simulink model "APP_MyApplication"  (R2018b)
settings: Solver=VariableStepDiscrete  StartTime=0.0  StopTime=10  RelTol=1e-3
PreLoadFcn:
  | if(exist('MBDS_ModelCallback', 'file')), MBDS_ModelCallback('PreLoad'); end;
PostLoadFcn:
  | if(exist('MBDS_ModelCallback', 'file')), MBDS_ModelCallback('PostLoad'); end;
InitFcn:
  | if(exist('MBDS_ModelCallback', 'file')), MBDS_ModelCallback('Init'); end;
StartFcn:
  | if(exist('MBDS_ModelCallback', 'file')), MBDS_ModelCallback('Start'); end;
StopFcn:
  | if(exist('MBDS_ModelCallback', 'file')), MBDS_ModelCallback('Stop'); end;
undefined symbols (not defined in the file): sigbuilder_block, Ts
libraries: KIBES_Signal x499, simulink x8
(part 1 of 10)
PreSaveFcn:
  | if(exist('MBDS_ModelCallback', 'file')), MBDS_ModelCallback('PreSave'); end;
CloseFcn:
  | if(exist('MBDS_ModelCallback', 'file')), MBDS_ModelCallback('Close'); end;
Description:
  | Design model of an MBDS Application
settings Model: IsTargetCode=true  MBDS_Version=08.20  Creator=Udo Kaiser (uidf0608)  LastModifiedBy=uidj2473
settings ConfigSet: Description=MBDS configuration set optimized for simulation of model designs for automotive embedded systems.
settings SolverCC: MinimalZcImpactIntegration=on
settings DataIOCC: MaxDataPoints=100  SaveFormat=StructureWithTime  SaveOutput=off  DSMLogging=off  VisualizeSimOutput=off  SaveTime=off  SignalLoggingName=LogSignals
settings OptimizationCC: UseDivisionForNetSlopeComputation=UseDivisionForReciprocalsOfIntegersOnly  UseFloatMulNetSlope=on  DefaultUnderspecifiedDataType=single  OptimizeBlockIOStorage=off  BufferReuse=off  GlobalBufferReuse=off  StrengthReduction=on  ExpressionFolding=off  ExpressionDepthLimit=2147483647  LocalBlockOutputs=off  EfficientFloat2IntCast=on  LifeSpan=inf  BufferReusableBoundary=off  OptimizeBlockOrder=speed  OptimizeDataStoreBuffers=off  BusAssignmentInplaceUpdate=off  LabelGuidedReuse=on
settings DebuggingCC: SignalInfNanChecking=error  AlgebraicLoopMsg=error  ArtificialAlgebraicLoopMsg=error  UnderspecifiedInitializationDetection=Classic  CheckExecutionContextPreStartOutputMsg=on  CheckExecutionContextRuntimeOutputMsg=on  BlockPriorityViolationMsg=error  MinStepSizeMsg=error  TimeAdjustmentMsg=warning  SolverPrmCheckMsg=error  InheritedTsInSrcMsg=none  SingleTaskRateTransMsg=error  TasksWithSamePriorityMsg=error  SigSpecEnsureSampleTimeMsg=error  CheckMatrixSingularityMsg=error  ParameterUnderflowMsg=error  ParameterTunabilityLossMsg=error  FixptConstUnderflowMsg=warning  FixptConstOverflowMsg=warning  FixptConstPrecisionLossMsg=warning  VectorMatrixConversionMsg=error  SignalLabelMismatchMsg=warning  SFcnCompatibilityMsg=error  FrameProcessingCompatibilityMsg=warning  UniqueDataStoreMsg=error  BusObjectLabelMismatch=error  RootOutportRequireBusObject=error  AllowSymbolicDim=off  ModelReferenceIOMsg=error  ModelReferenceIOMismatchMessage=error  UnknownTsInhSupMsg=error  ModelReferenceDataLoggingMessage=error  StateNameClashWarn=warning  SimStateOlderReleaseMsg=warning  StrictBusMsg=ErrorOnBusTreatedAsVector  NonBusSignalsTreatedAsBus=error  SFInvalidInputDataAccessInChartInitDiag=error  SFTransitionOutsideNaturalParentDiag=error  SFUnreachableExecutionPathDiag=error  SFUndirectedBroadcastEventsDiag=error  SFTransitionActionBeforeConditionDiag=error  SFTemporalDelaySmallerThanSampleTimeDiag=error  SFExecutionAtInitializationDiag=none
settings HardwareCC: ProdBitPerPointer=32  ProdBitPerSizeT=32  ProdBitPerPtrDiffT=32  ProdLargestAtomicInteger=Long  ProdEndianess=BigEndian  ProdWordSize=32  ProdLongLongMode=on  ProdHWDeviceType=Custom Processor  TargetHWDeviceType=32-bit Generic
settings ModelReferenceCC: PropagateSignalLabelsOutOfModel=off
settings SFSimCC: SimUseLocalCustomCode=off  SimGenImportedTypeDefs=on  CompileTimeRecursionLimit=0  EnableRuntimeRecursion=off  MATLABDynamicMemAlloc=off  DefaultCustomCodeFunctionArrayLayout=Column-major
settings RTWCC: SystemTargetFile=MBDS.tlc  GenCodeOnly=on  TemplateMakefile=MBDS.tmf  Description=MBDS Target  GenerateReport=on  RTWUseLocalCustomCode=off  IncludeHyperlinkInReport=on  LaunchReport=on  GenerateTraceReport=on  GenerateTraceReportSl=on  GenerateTraceReportSf=on  GenerateTraceReportEml=on  GenerateCodeMetricsReport=on  RTWCompilerOptimization=on
settings CodeAppCC: ForceParamTrailComments=on  IgnoreCustomStorageClasses=off  OperatorAnnotations=on  SimulinkDataObjDesc=on  SFDataObjDesc=on  MangleLength=2  CustomSymbolStrType=$N$R$M  CustomSymbolStrFcn=$R$M  CustomSymbolStrUtil=$n$C  InsertBlockDesc=on  StateflowObjectComments=on  MATLABSourceComments=on  ReqsInCode=on  UseSimReservedNames=on
settings STFCustomTargetCC: UtilityFuncGeneration=Shared location  MultiwordLength=256  DynamicStringBufferSize=2  InferredTypesCompatibility=on  ModelReferenceCompliant=off  IncludeMdlTerminateFcn=off  CombineOutputUpdateFcns=on  CombineSignalStateStructs=on  SuppressErrorStatus=on  ERTCustomFileBanners=on  SupportComplex=off  SupportContinuousTime=off  SupportNonInlinedSFcns=off  RemoveDisableFunc=on  RemoveResetFunc=on  ParenthesesLevel=Maximum  CastingMode=Standards  MATLABClassNameForMDSCustomization=Simulink.SoftwareTarget.ERTCustomization  GenerateSharedConstants=off  SystemTargetFile=MBDS.tlc
settings ERTTargetCC: UtilityFuncGeneration=Shared location  DynamicStringBufferSize=2  InferredTypesCompatibility=on  ModelReferenceCompliant=off  ParMdlRefBuildCompliant=off  CompOptLevelCompliant=off  ConcurrentExecutionCompliant=off  IncludeMdlTerminateFcn=off  CombineSignalStateStructs=on  SuppressErrorStatus=on  SupportComplex=off  RemoveDisableFunc=on  ParenthesesLevel=Maximum  CastingMode=Standards  ModelStepFunctionPrototypeControlCompliant=off  CPPClassGenCompliant=off  UseToolchainInfoCompliant=off  GenerateSharedConstants=off  ERTCustomFileTemplate=example_file_process.tlc  EnableDataOwnership=on  PreserveExpressionOrder=on  PreserveIfCondition=on  SuppressUnreachableDefaultCases=off  EnableSignedLeftShifts=off  EnableSignedRightShifts=off  IndentStyle=Allman  NewlineStyle=CR+LF
settings ConfigComp: CovScope=ReferencedModels  CovIncludeTopModel=off  CovPath=APP_MyApplication/Model/APP_MyApplication_  CovSaveName=covData  CovMetricSettings=dsw  CovFilter=MBDS_CoverageFilter  CovHTMLOptions=-sRT=1 -sVT=0 -aTS=1 -bRG=1 -bTC=1 -hTR=1 -nFC=0 -nFD=0 -scm=1 -bcm=1 -xEv=0 -xEM=1  CovHtmlReporting=on  CovSaveOutputData=off  CovDataFileName=covData  CovShowResultsExplorer=off  CovExternalEMLEnable=off  CovSFcnEnable=off

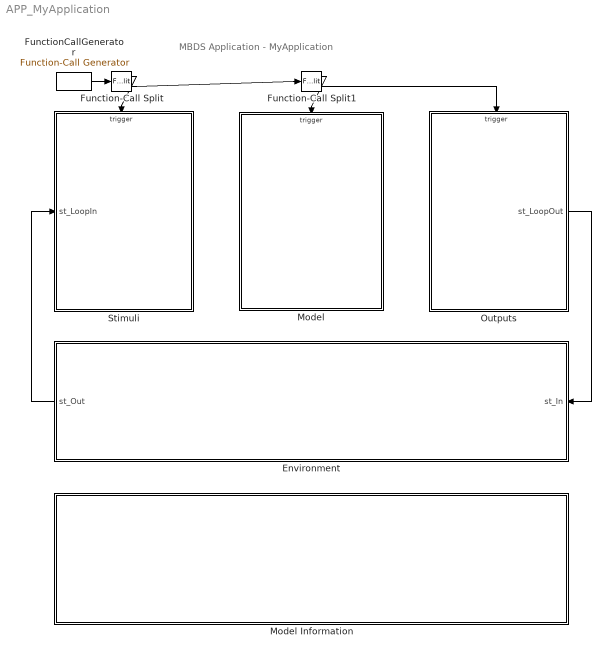
== system APP_MyApplication ==
  note: MBDS Application - MyApplication
  Environment : Subsystem  Description=Environment subsystem for a MBDS model.
  Function-Call Split : FunctionCallSplit  InitFcn=|  NumOutputPorts=2
      | try
      |    MBDS_BlockCallback('Update', gcb);
      | end
      | try
      |    MBDS_BlockCallback('Update', gcb);
      | end
  Function-Call Split1 : FunctionCallSplit  InitFcn=|  NumOutputPorts=2
      | try
      |    MBDS_BlockCallback('Update', gcb);
      | end
      | try
      |    MBDS_BlockCallback('Update', gcb);
      | end
  FunctionCallGenerator : simulink/Ports & Subsystems/Function-Call Generator  sample_time=0.05  numberOfIterations=1
      settings: AttributesFormatString=Ts = %<sample_time>
  Model : Subsystem  Description=Model subsystem for a MBDS model. Here, the input signals to the model functionality are resolved from the Stimuli bus and the output signals of the model functionality are summarized into the Results bus.
  Model Information : Subsystem  InitFcn=|  mask(ModelInformation){MBDS_LibraryBlock=on, Company=-, Department=-, Responsible=-, Status=In Work, Complete=on, Check=on, Test=on, Optimize=on, Documentation=on, FcnErrors=off, GenericToDo=off, DocumentState=Draft, GenericToDoName=Enter a user specific ToDo text, MBDS_BlockVersion=07.00}
      | if(exist('MBDS_BlockCallback', 'file'))
      |    MBDS_BlockCallback('Update', gcb);
      | end
      mask prompts: MBDS_LibraryBlock "MBDS Library Block"; Complete "Complete Implementation"; Check "Check Modelling Guidelines"; Test "Test Functionality"; Optimize "Optimize Implementation"; Documentation "Create Documentation"; FcnErrors "Remove Functional Errors"; GenericToDo "Enter a user specific ToDo text"; DocumentState "Document State:"; GenericToDoName "Generic ToDo Name:"; MBDS_BlockVersion "Block version:"
      mask help: This block displays model information and ToDo's on it's block mask. Via the block parameter mask further model information and configuration options can be accessed.
      mask init:
      | if(exist('MBDS_BlockCallback', 'file'))
      |    MBDS_BlockCallback('Copy', gcb);    
      | end
      mask Help: eval(['open([workdir(''library_dir:''),''\Blockset\help\'',get_param(gcb,''MaskType''),''.html''])'])
      mask TypeOptions Status: In Work | Done
      mask TypeOptions DocumentState: Draft | Final | Released
      mask Callback GenericToDoName:
      | MaskPrompts = get_param(gcb, 'MaskPrompts');
      | MaskPrompts{12} = get_param(gcb, 'GenericToDoName');
      | if(length(MaskPrompts{12}) > 75)
      |    MaskPrompts{12} = MaskPrompts{12}(1:75);
      |    set_param(gcb, 'GenericToDoName', MaskPrompts{12});
      | end
      | set_param(gcb, 'MaskPrompts', MaskPrompts);
      | clear MaskPrompts;
      mask DialogControl ParameterTabVar0 Prompt: Info
      mask DialogControl ParameterTabVar01 Prompt: ToDo's
      mask DialogControl ParameterTabVar012 Prompt: Options
      mask DialogControl ParameterTabVar0123 Prompt: Version
      mask Display:
      | % Get ToDo's
      | IsComplete       = strcmpi(Complete, 'on');
      | IsOptimize       = strcmpi(Optimize, 'on');
      | IsCheck          = strcmpi(Check, 'on');
      | IsDocumentation  = strcmpi(Documentation, 'on');
      | IsTest           = strcmpi(Test, 'on');
      | IsFcnErrors      = strcmpi(FcnErrors, 'on');
      | IsGenericToDo    = strcmpi(GenericToDo, 'on');
      | 
      | % Determine status
      | if(IsFcnErrors || IsTest || IsComplete || IsDocumentation || IsCheck || IsOptimize || IsGenericToDo)
      |    Status = 'In Work';
      | else
      |    Status = 'Done';
      | end
      | 
      | % Update status parameter
      | if(~strcmpi(get_param(gcb, 'Status'), Status))
      |    set_param(gcb, 'Status', Status);
      | end
      | 
      | % Determine severity
      | if(IsFcnErrors)
      |    % Severity: Critical
      |    BoxColorFile = 'Box_Red.tif';
      |    IconFile     = 'State_Red.jpg';
      | elseif (IsTest || IsComplete || IsGenericToDo)
      |    % Severity: Major
      |    BoxColorFile = 'Box_Orange.tif';
      |    IconFile     = 'State_Orange.jpg';
      | elseif (IsDocumentation || IsCheck || IsOptimize)
      |    % Severity: Minor
      |    BoxColorFile = 'Box_Grey.tif';
      |    IconFile     = 'State_Grey.jpg';
      | else
      |    % Severity: None
      |    BoxColorFile = 'Box_Green.tif';
      |    IconFile     = 'State_Green.jpg';
      | end
      | 
      | % Display Model Information
      | InfoStr1 = sprintf('%s', get_param(bdroot, 'Name'));
      | InfoStr2 = sprintf('Model Version:  %s', get_param(bdroot, 'ModelVersion'));
      | InfoStr3 = sprintf('Company:  %s', Company);
      | InfoStr4 = sprintf('Department:  %s', Department);
      | InfoStr5 = sprintf('Responsible:  %s', Responsible);
      | InfoStr6 = sprintf('Last Modified by:  %s at %s', get_param(bdroot, 'LastModifiedBy'), get_param(bdroot, 'LastModifiedDate'));
      | %Y is to do!!!!
      | text(0.5, 0.69, sprintf('%s\n%s\n%s\n%s\n%s\n%s\n%s', InfoStr1, InfoStr2, InfoStr3, InfoStr4, InfoStr5, InfoStr6), 'horizontalAlignment', 'center');
      | clear InfoStr1 InfoStr2 InfoStr3 InfoStr4 InfoStr5 InfoStr6;
      | 
      | % Display Status
      | if(exist(BoxColorFile, 'file'))
      |    image(imread(BoxColorFile,'tif'), [0,0,1,0.45]);
      | end
      | if(exist(IconFile, 'file'))
      |    image(imread(IconFile,'jpg'), [0.025,0.09,0.08,0.26]);
      |    image(imread(IconFile,'jpg'), [0.9,0.09,0.08,0.26]);
      | end
      | plot([-0.01 1.01], [0.45 0.45])
      | text(0.5, 0.38, sprintf('Status: %s', upper(Status)), 'horizontalAlignment', 'center');
      | 
      | % Display ToDo's
      | if(IsComplete)
      |    text(0.15, 0.31, '- Complete Implementation');
      | end
      | if(IsOptimize)
      |    text(0.6, 0.31, '- Optimize Implementation');
      | end
      | 
      | if(IsCheck)
      |    text(0.15, 0.23, '- Check Modeling Guidelines');
      | end
      | if(IsDocumentation)
      |    text(0.6, 0.23, '- Create Documentation');
      | end
      | 
      | if(IsTest)
      |    text(0.15, 0.14, '- Test Functionality');
      | end
      | if(IsFcnErrors)
      |    text(0.6, 0.14, '- Remove Functional Errors');
      | end
      | 
      | if(IsGenericToDo)
      |    text(0.15, 0.06, ['- ', GenericToDoName]);
      | end
  Outputs : Subsystem  Description=Result subsystem for a MBDS model. Here, output signals from the model functionality can be displayed using a scope or display. Additionally, the output signals can be postprocessed before they will passed to the feedback loop.
  Stimuli : Subsystem  Description=Stimuli subsystem for a MBDS model. Here, input signals for testing the model functionality can be defined using the signal builder or calculated applying arbitrary basic-blocks. Additionally, feedback signals can be preprocessed at this stage.
  wires:
  Outputs/1(st_LoopOut) -> Environment/1(st_In)
  Environment/1(st_Out) -> Stimuli/1(st_LoopIn)
  FunctionCallGenerator/1 -> Function-Call Split/1
  Function-Call Split/1 -> Stimuli/Trigger
  Function-Call Split1/2 -> Outputs/Trigger
  Function-Call Split1/1 -> Model/Trigger
  Function-Call Split/2 -> Function-Call Split1/1

== system APP_MyApplication/Environment ==
  st_In : Inport
  Bus_Creator : BusCreator  InitFcn=|  Inputs=2
      | try
      |    MBDS_BlockCallback('Update', gcb);
      | end
      | try
      |    MBDS_BlockCallback('Update', gcb);
      | end
  Bus_Selector : BusSelector  InitFcn=|  OutputSignals=bo_Out1,i32_Out2
      | try
      |    MBDS_BlockCallback('Update', gcb);
      | end
      | try
      |    MBDS_BlockCallback('Update', gcb);
      | end
  Ground : Ground  InitFcn=|
      | try
      |    MBDS_BlockCallback('Update', gcb);
      | end
  Ground1 : Ground  InitFcn=|
      | try
      |    MBDS_BlockCallback('Update', gcb);
      | end
  Rate Transition1 : RateTransition  InitFcn=|  OutPortSampleTimeOpt=Inherit
      | try
      |    MBDS_BlockCallback('Update', gcb);
      | end
  Rate Transition3 : RateTransition  InitFcn=|  OutPortSampleTimeOpt=Inherit
      | try
      |    MBDS_BlockCallback('Update', gcb);
      | end
  Terminator : Terminator
      settings: InitFcn=|
      | try
      |    MBDS_BlockCallback('Update', gcb);
      | end
  Terminator1 : Terminator
      settings: InitFcn=|
      | try
      |    MBDS_BlockCallback('Update', gcb);
      | end
  Unit_Delay : UnitDelay  InitFcn=|  SampleTime=-1
      | try
      |    MBDS_BlockCallback('Update', gcb);
      | end
      | try                                  
      |    MBDS_BlockCallback('Update', gcb);
      | end
      settings: AttributesFormatString=Init = %<X0>
  st_Out : Outport
  wires:
  Bus_Creator/1 -> Rate Transition3/1
  Bus_Selector/1 -> Terminator/1  "<bo_Out1>"
  Ground/1 -> Bus_Creator/1  "d_Feedback1"
  Ground1/1 -> Bus_Creator/2  "d_Feedback2"
  Bus_Selector/2 -> Terminator1/1  "<i32_Out2>"
  Unit_Delay/1 -> Rate Transition1/1
  Rate Transition1/1 -> Bus_Selector/1
  Rate Transition3/1 -> st_Out/1  "st_Out"
  st_In/1 -> Unit_Delay/1

== system APP_MyApplication/Model ==
  Function : TriggerPort  InitFcn=|  TriggerType=function-call  VariantControl=(inherit)
      | try
      |    MBDS_BlockCallback('Update', gcb);
      | end
  APP_MyApplication_ : Subsystem  Tag=Functionality
      settings: AttributesFormatString=Functionality

== system APP_MyApplication/Model Information ==
  note: Double Click the Model Information block to open the block parameter mask

== system APP_MyApplication/Outputs ==
  note: Specify Reference Signals
  note: Return outputs from ECU-Signals
      | by using Virtual Connector Blocks
  Function : TriggerPort  InitFcn=|  TriggerType=function-call  VariantControl=(inherit)
      | try
      |    MBDS_BlockCallback('Update', gcb);
      | end
  AnalyseOutputs : Subsystem
  Assertion : Assertion  Enabled=off
  Bus_Selector : BusSelector  InitFcn=|  OutputSignals=bo_Out1,i32_Out2
      | try
      |    MBDS_BlockCallback('Update', gcb);
      | end
      | try
      |    MBDS_BlockCallback('Update', gcb);
      | end
  Data Type Conversion1 : DataTypeConversion  InitFcn=|  OutDataTypeStr=int32
      | try
      |    MBDS_BlockCallback('Update', gcb);
      | end
      | try
      |    MBDS_BlockCallback('Update', gcb);
      | end
  Data Type Conversion3 : DataTypeConversion  InitFcn=|  OutDataTypeStr=boolean
      | try
      |    MBDS_BlockCallback('Update', gcb);
      | end
      | try
      |    MBDS_BlockCallback('Update', gcb);
      | end
  Ground1 : Ground  InitFcn=|
      | try
      |    MBDS_BlockCallback('Update', gcb);
      | end
      | try
      |    MBDS_BlockCallback('Update', gcb);
      | end
  Ground2 : Ground  InitFcn=|
      | try
      |    MBDS_BlockCallback('Update', gcb);
      | end
      | try
      |    MBDS_BlockCallback('Update', gcb);
      | end
  Outputs : Scope  NumInputPorts=2
  OutputsBusCreator : BusCreator  InitFcn=|  Inputs=2
      | try
      |    MBDS_BlockCallback('Update', gcb);
      | end
      | try
      |    MBDS_BlockCallback('Update', gcb);
      | end
  References : Subsystem  Tag=STV Subsys  LoadFcn=sigbuilder_block('load');  StartFcn=sigbuilder_block('start');  StopFcn=sigbuilder_block('stop');  ClipboardFcn=sigbuilder_block('clipboard');  mask(Sigbuilder block){tuvar=[0:10]}
      mask help: Sigbuilder GUI
      mask init:
      | if ~strcmp(get_param(bdroot(gcbh),'SimulationStatus'),'stopped') tuvar = sigbuilder_block('maskInit'); end
      settings: CopyFcn=sigbuilder_block('copy');  DeleteFcn=sigbuilder_block('delete');  ModelCloseFcn=sigbuilder_block('modelClose');  PreSaveFcn=sigbuilder_block('preSave');  PauseFcn=sigbuilder_block('pause')  ContinueFcn=sigbuilder_block('continue')  NameChangeFcn=sigbuilder_block('namechange');  OpenFcn=sigbuilder_block('open',[248.25 204 550.5 399.75 ]);  CloseFcn=sigbuilder_block('close');
      mask Display: plot(0, 0, 100, 100,[2, 2, 32, 32, 2], [68, 8, 8, 68, 68],[32, 2], [38, 38], [32, 19, 2],[53, 60, 44], [32, 17, 17, 2],[16, 16, 31, 31]);txt = getActiveGroup(gcbh);text(2, 100, txt,'verticalAlignment', 'top');
  ReferencesBusCreator : BusCreator  InitFcn=|  Inputs=2
      | try
      |    MBDS_BlockCallback('Update', gcb);
      | end
      | try
      |    MBDS_BlockCallback('Update', gcb);
      | end
  Signal Conversion : SignalConversion  InitFcn=|  OverrideOpt=off
      | try
      |    MBDS_BlockCallback('Update', gcb);
      | end
  st_LoopOut : Outport
  wires:
  Bus_Selector/1 -> Outputs/1  "<bo_Out1>"
  Bus_Selector/2 -> Outputs/2  "<i32_Out2>"
  Data Type Conversion3/1 -> ReferencesBusCreator/1  "bo_Out1_Ref"
  Data Type Conversion1/1 -> ReferencesBusCreator/2  "i32_Out2_Ref"
  ReferencesBusCreator/1 -> AnalyseOutputs/2(st_References)  "st_References"
  AnalyseOutputs/1(bo_IsOutputValid) -> Assertion/1
  Ground2/1 -> OutputsBusCreator/2  "i32_Out2"
  OutputsBusCreator/1 -> Signal Conversion/1, Bus_Selector/1, AnalyseOutputs/1(st_Outputs)  "st_Outputs"
  Ground1/1 -> OutputsBusCreator/1  "bo_Out1"
  References/1(bo_Out1_Ref) -> Data Type Conversion3/1
  References/2(i32_Out2_Ref) -> Data Type Conversion1/1
  Signal Conversion/1 -> st_LoopOut/1  "st_LoopOut"

== system APP_MyApplication/Stimuli ==
  note: Specifiy Stimuli
  note: Feed Stimuli to ECU-Signals
      | by using Virtual Connector Blocks
  note: For closed-loop simulations use feedback signals
      | from environment subsystem as model stimuli
  st_LoopIn : Inport
      settings: LatchInputForFeedbackSignals=on
  Function : TriggerPort  InitFcn=|  TriggerType=function-call  VariantControl=(inherit)
      | try
      |    MBDS_BlockCallback('Update', gcb);
      | end
  Bus_Selector : BusSelector  InitFcn=|  OutputSignals=d_Feedback1,d_Feedback2
      | try
      |    MBDS_BlockCallback('Update', gcb);
      | end
      | try
      |    MBDS_BlockCallback('Update', gcb);
      | end
  Bus_Selector1 : BusSelector  InitFcn=|  OutputSignals=bo_In1,i32_In2
      | try
      |    MBDS_BlockCallback('Update', gcb);
      | end
      | try
      |    MBDS_BlockCallback('Update', gcb);
      | end
  Data Type Conversion1 : DataTypeConversion  InitFcn=|  OutDataTypeStr=int32
      | try
      |    MBDS_BlockCallback('Update', gcb);
      | end
      | try
      |    MBDS_BlockCallback('Update', gcb);
      | end
  Data Type Conversion3 : DataTypeConversion  InitFcn=|  OutDataTypeStr=boolean
      | try
      |    MBDS_BlockCallback('Update', gcb);
      | end
      | try
      |    MBDS_BlockCallback('Update', gcb);
      | end
  Stimuli : Subsystem  Tag=STV Subsys  LoadFcn=sigbuilder_block('load');  StartFcn=sigbuilder_block('start');  StopFcn=sigbuilder_block('stop');  ClipboardFcn=sigbuilder_block('clipboard');  mask(Sigbuilder block){tuvar=[0:10]}
      mask help: Sigbuilder GUI
      mask init:
      | if ~strcmp(get_param(bdroot(gcbh),'SimulationStatus'),'stopped') tuvar = sigbuilder_block('maskInit'); end
      settings: CopyFcn=sigbuilder_block('copy');  DeleteFcn=sigbuilder_block('delete');  ModelCloseFcn=sigbuilder_block('modelClose');  PreSaveFcn=sigbuilder_block('preSave');  PauseFcn=sigbuilder_block('pause')  ContinueFcn=sigbuilder_block('continue')  NameChangeFcn=sigbuilder_block('namechange');  OpenFcn=sigbuilder_block('open',[190.5 198 550.5 399.75 ]);  CloseFcn=sigbuilder_block('close');
      mask Display: plot(0, 0, 100, 100,[2, 2, 32, 32, 2], [68, 8, 8, 68, 68],[32, 2], [38, 38], [32, 19, 2],[53, 60, 44], [32, 17, 17, 2],[16, 16, 31, 31]);txt = getActiveGroup(gcbh);text(2, 100, txt,'verticalAlignment', 'top');
  StimuliBusCreator : BusCreator  InitFcn=|  Inputs=2
      | try
      |    MBDS_BlockCallback('Update', gcb);
      | end
      | try
      |    MBDS_BlockCallback('Update', gcb);
      | end
  Terminator{,1..3} (4 alike) : Terminator
      settings: InitFcn=|
      | try
      |    MBDS_BlockCallback('Update', gcb);
      | end
      | try
      |    MBDS_BlockCallback('Update', gcb);
      | end
  wires:
  Bus_Selector/1 -> Terminator/1  "<d_Feedback1>"
  Bus_Selector/2 -> Terminator1/1  "<d_Feedback2>"
  Stimuli/1(bo_In1) -> Data Type Conversion3/1
  Stimuli/2(i32_In2) -> Data Type Conversion1/1
  StimuliBusCreator/1 -> Bus_Selector1/1  "st_Stimuli"
  Data Type Conversion3/1 -> StimuliBusCreator/1  "bo_In1"
  Data Type Conversion1/1 -> StimuliBusCreator/2  "i32_In2"
  Bus_Selector1/1 -> Terminator2/1  "<bo_In1>"
  Bus_Selector1/2 -> Terminator3/1  "<i32_In2>"
  st_LoopIn/1 -> Bus_Selector/1

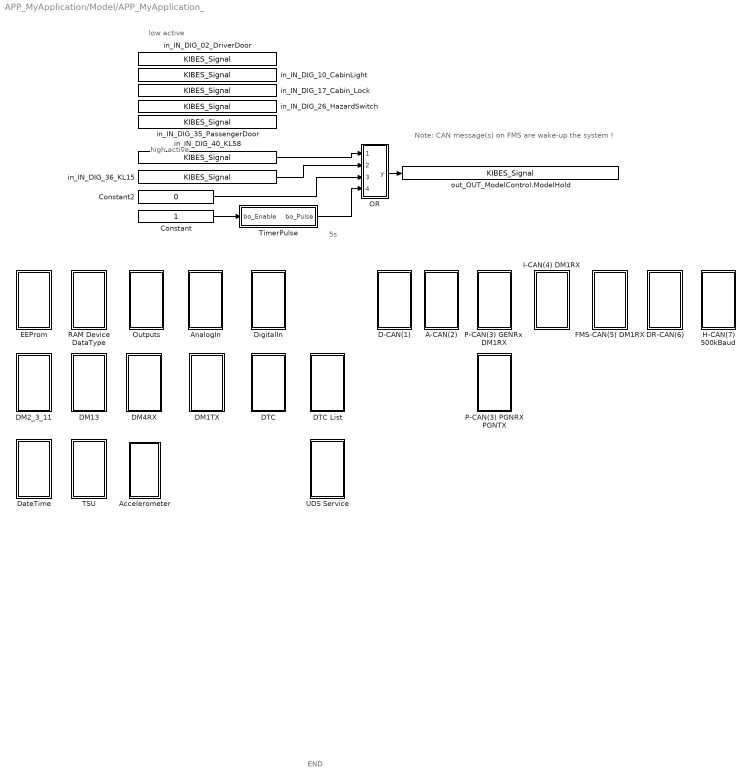
== system APP_MyApplication/Model/APP_MyApplication_ ==
  note: END
  note: high active
  note: low active
  note: Note: CAN message(s) on FMS are wake-up the system !
  note: 5s
  A-CAN(2) : Subsystem
  "Accelerometer " : Subsystem
  AnalogIn : Subsystem
  Constant : Constant  InitFcn=|  OutDataTypeStr=boolean
      | if(exist('MBDS_BlockCallback', 'file'))
      |    MBDS_BlockCallback('Update', gcb);  
      | end
  Constant2 : Constant  InitFcn=|  Value=0  OutDataTypeStr=boolean
      | if(exist('MBDS_BlockCallback', 'file'))
      |    MBDS_BlockCallback('Update', gcb);  
      | end
  D-CAN(1) : Subsystem
  DM13 : Subsystem
  DM1TX : Subsystem
  DM2_3_11 : Subsystem
  DM4RX : Subsystem
  DR-CAN(6) : Subsystem
  DTC : Subsystem
  DTC List : Subsystem
  DateTime : Subsystem
  DigitalIn : Subsystem
  EEProm : Subsystem
  FMS-CAN(5) DM1RX : Subsystem
  H-CAN(7) 500kBaud : Subsystem
  I-CAN(4) DM1RX : Subsystem
  OR : Subsystem  InitFcn=|  mask(OR){MBDS_LibraryBlock=on, BitwiseMode=off, Inputs=4, UseBitMask=off, BitMask='A1', OutDataTypeStr=Inherit: Inherit via back propagation, MBDS_BlockVersion=07.21.05}
      | if(exist('MBDS_BlockCallback', 'file'))
      |    MBDS_BlockCallback('Update', gcb);
      | end
      mask prompts: MBDS_LibraryBlock "MBDS library block"; BitwiseMode "Use 'bitwise' mode"; Inputs "Number of input ports:"; UseBitMask "Use bit mask"; BitMask "Bit mask:"; OutDataTypeStr "Output data type:"; MBDS_BlockVersion "Version:"
      mask help: Logical or bitwise OR operator. For multiple inputs, operators are applied across the inputs. For a single input, operators are applied across the input vector. In bitwise mode a bit mask can be applied onto single input signals.
      mask init:
      | if(exist('MBDS_BlockCallback', 'file'))
      |    MBDS_BlockCallback('Init', gcb);
      | else
      |    % Disable all mask parameters
      |    MaskEnables = get_param(gcb, 'MaskEnables');
      |    for k = [1:length(MaskEnables)]
      |       MaskEnables{k} = 'off';
      |    end
      |    if(~isequal(MaskEnables, get_param(gcb, 'MaskEnables')))
      |       set_param(gcb, 'MaskEnables', MaskEnables);
      |    end
      | end
      mask Help: eval(['open([workdir(''library_dir:''),''\Blockset\help\'',get_param(gcb,''MaskType''),''.html''])'])
      mask Callback BitwiseMode:
      | if(exist('MBDS_BlockCallback', 'file'))
      |    MBDS_BlockCallback('BitwiseMode', gcb);
      | end
      mask Callback Inputs:
      | if(exist('MBDS_BlockCallback', 'file'))
      |    MBDS_BlockCallback('Inputs', gcb);
      | end
      mask Callback UseBitMask:
      | if(exist('MBDS_BlockCallback', 'file'))
      |    MBDS_BlockCallback('UseBitMask', gcb);
      | end
      mask Callback BitMask:
      | if(exist('MBDS_BlockCallback', 'file'))
      |    MBDS_BlockCallback('BitMask', gcb);
      | end
      mask TypeOptions OutDataTypeStr: Inherit: Inherit via back propagation | int8 | uint8 | int16 | uint16 | int32 | uint32 | boolean
      mask Callback OutDataTypeStr:
      | % Adopt Value
      | if(exist('MBDS_BlockCallback', 'file'))
      |    MBDS_BlockCallback('OutDataTypeStr', gcb);
      | end
      mask DialogControl ParameterTabVar0 Prompt: Main
      mask DialogControl ParameterTabVar01 Prompt: Signal Attributes
      mask DialogControl ParameterTabVar012 Prompt: Version
      mask Display:
      | % Show icon or block text
      | if(UseBitMask)
      |    if(isnumeric(BitMask))
      |       BitMaskString = ['0x',dec2hex(floor(BitMask))];
      |    elseif(ischar(BitMask))
      |       BitMaskString = ['0x',upper(BitMask)];
      |    else
      |       BitMaskString = '???';
      |    end
      |    disp(sprintf(['OR\n', BitMaskString]))
      | else
      |    disp('OR')
      | end
  Outputs : Subsystem
  P-CAN(3) GENRx  DM1RX : Subsystem
  P-CAN(3) PGNRX PGNTX : Subsystem
  RAM Device DataType : Subsystem
  TSU : Subsystem
  TimerPulse : Subsystem
  UDS Service : Subsystem
  in_IN_DIG_02_DriverDoor : KIBES_Signal/KIBES_Signal  MBDS_LibraryBlock=on  DatabaseKey=215  SignalName=IN_DIG_02_DriverDoor  SymbolName=IN_DIG_02_DriverDoor_000215  DataType=boolean  Init=0  Slope=1  Bias=0  DataSize=1  fpDataType=boolean  BlockIOType=Inport  DeviceType=0
  in_IN_DIG_10_CabinLight : KIBES_Signal/KIBES_Signal  MBDS_LibraryBlock=on  DatabaseKey=213  SignalName=IN_DIG_10_CabinLight  SymbolName=IN_DIG_10_CabinLight_000213  DataType=boolean  Init=0  Slope=1  Bias=0  DataSize=1  fpDataType=boolean  BlockIOType=Inport  DeviceType=0
  in_IN_DIG_17_Cabin_Lock : KIBES_Signal/KIBES_Signal  MBDS_LibraryBlock=on  DatabaseKey=211  SignalName=IN_DIG_17_Cabin_Lock  SymbolName=IN_DIG_17_Cabin_Lock_000211  DataType=boolean  Init=0  Slope=1  Bias=0  DataSize=1  fpDataType=boolean  BlockIOType=Inport  DeviceType=0
  in_IN_DIG_26_HazardSwitch : KIBES_Signal/KIBES_Signal  MBDS_LibraryBlock=on  DatabaseKey=212  SignalName=IN_DIG_26_HazardSwitch  SymbolName=IN_DIG_26_HazardSwitch_000212  DataType=boolean  Init=0  Slope=1  Bias=0  DataSize=1  fpDataType=boolean  BlockIOType=Inport  DeviceType=0
  in_IN_DIG_35_PassengerDoor : KIBES_Signal/KIBES_Signal  MBDS_LibraryBlock=on  DatabaseKey=214  SignalName=IN_DIG_35_PassengerDoor  SymbolName=IN_DIG_35_PassengerDoor_000214  DataType=boolean  Init=0  Slope=1  Bias=0  DataSize=1  fpDataType=boolean  BlockIOType=Inport  DeviceType=0
  in_IN_DIG_36_KL15 : KIBES_Signal/KIBES_Signal  MBDS_LibraryBlock=on  DatabaseKey=216  SignalName=IN_DIG_36_KL15  SymbolName=IN_DIG_36_KL15_000216  DataType=boolean  Init=0  Slope=1  Bias=0  DataSize=1  fpDataType=boolean  BlockIOType=Inport  DeviceType=0
  in_IN_DIG_40_KL58 : KIBES_Signal/KIBES_Signal  MBDS_LibraryBlock=on  DatabaseKey=210  SignalName=IN_DIG_40_KL58  SymbolName=IN_DIG_40_KL58_000210  DataType=boolean  Init=0  Slope=1  Bias=0  DataSize=1  fpDataType=boolean  BlockIOType=Inport  DeviceType=0
  out_OUT_ModelControl.ModelHold : KIBES_Signal/KIBES_Signal  MBDS_LibraryBlock=on  DatabaseKey=1  SignalName=OUT_ModelControl.ModelHold  SymbolName=OUT_ModelControl_ModelHold_000001  DataType=boolean  Init=0  Slope=1  Bias=0  DataSize=1  fpDataType=boolean  BlockIOType=Outport  DeviceType=0
  wires:
  in_IN_DIG_40_KL58/1 -> OR/1(u1)
  OR/1(y) -> out_OUT_ModelControl.ModelHold/1
  in_IN_DIG_36_KL15/1 -> OR/2(u2)
  Constant2/1 -> OR/3(u3)
  TimerPulse/1(bo_Pulse) -> OR/4(u4)
  Constant/1 -> TimerPulse/1(bo_Enable)

== system APP_MyApplication/Outputs/AnalyseOutputs ==
  note: Compare Output- with Reference-Signals
      | -----------------------------------------------------------------
      | - Modify this subsystem according to your needs
      | -  Use Assertion blocks of the MBDS Standard Library for automatic inspection
      | - Use arithmetic and logical blocks for analysing errors
  st_Outputs : Inport  InitFcn=|
      | try
      |    MBDS_BlockCallback('Update', gcb);
      | end
  st_References : Inport  InitFcn=|  Port=2
      | try
      |    MBDS_BlockCallback('Update', gcb);
      | end
  AND : Subsystem  InitFcn=|  mask(AND){MBDS_LibraryBlock=on, BitwiseMode=off, Inputs=2, UseBitMask=off, BitMask=0, OutDataTypeStr=Inherit: Inherit via back propagation, MBDS_BlockVersion=05.20}
      | if(exist('MBDS_BlockCallback', 'file'))
      |    MBDS_BlockCallback('Update', gcb);
      | end
      mask prompts: MBDS_LibraryBlock "MBDS library block"; BitwiseMode "Use 'bitwise' mode"; Inputs "Number of input ports:"; UseBitMask "Use bit mask"; BitMask "Bit mask:"; OutDataTypeStr "Output data type:"; MBDS_BlockVersion "Version:"
      mask help: Logical or bitwise AND operator. For multiple inputs, operators are applied across the inputs. For a single input, operators are applied across the input vector. In bitwise mode a bit mask can be applied onto single input signals.
      mask init: same as APP_MyApplication/Model/APP_MyApplication_/OR
      mask Help: eval(['open([workdir(''library_dir:''),''\Blockset\help\'',get_param(gcb,''MaskType''),''.html''])'])
      mask Callback BitwiseMode:
      | if(exist('MBDS_BlockCallback', 'file'))
      |    MBDS_BlockCallback('BitwiseMode', gcb);
      | end
      mask Callback Inputs:
      | if(exist('MBDS_BlockCallback', 'file'))
      |    MBDS_BlockCallback('Inputs', gcb);
      | end
      mask Callback UseBitMask:
      | if(exist('MBDS_BlockCallback', 'file'))
      |    MBDS_BlockCallback('UseBitMask', gcb);
      | end
      mask Callback BitMask:
      | if(exist('MBDS_BlockCallback', 'file'))
      |    MBDS_BlockCallback('BitMask', gcb);
      | end
      mask TypeOptions OutDataTypeStr: Inherit: Inherit via back propagation | int8 | uint8 | int16 | uint16 | int32 | uint32 | boolean
      mask Callback OutDataTypeStr:
      | % Adopt Value
      | if(exist('MBDS_BlockCallback', 'file'))
      |    MBDS_BlockCallback('OutDataTypeStr', gcb);
      | end
      mask DialogControl ParameterTabVar0 Prompt: Main
      mask DialogControl ParameterTabVar01 Prompt: Signal Attributes
      mask DialogControl ParameterTabVar012 Prompt: Version
      mask Display:
      | % Show icon or block text
      | if(UseBitMask)
      |    if(isnumeric(BitMask))
      |       BitMaskString = ['0x',dec2hex(floor(BitMask))];
      |    elseif(ischar(BitMask))
      |       BitMaskString = ['0x',upper(BitMask)];
      |    else
      |       BitMaskString = '???';
      |    end
      |    disp(sprintf(['AND\n', BitMaskString]))
      | else
      |    disp('AND')
      | end
  Abs1 : Abs  InitFcn=|  OutDataTypeStr=Inherit: Inherit via back propagation
      | if(exist('MBDS_BlockCallback', 'file'))
      |    MBDS_BlockCallback('Update', gcb);  
      | end
      settings: AttributesFormatString=Saturate: %<SaturateOnIntegerOverflow>
  Abs2 : Abs  InitFcn=|  OutDataTypeStr=Inherit: Inherit via back propagation
      | if(exist('MBDS_BlockCallback', 'file'))
      |    MBDS_BlockCallback('Update', gcb);  
      | end
      settings: AttributesFormatString=Saturate: %<SaturateOnIntegerOverflow>
  Add : Sum  InitFcn=|  Inputs=+-  OutDataTypeStr=int32  SaturateOnIntegerOverflow=on  InputSameDT=on
      | if(exist('MBDS_BlockCallback', 'file'))
      |    MBDS_BlockCallback('Update', gcb);  
      | end
      settings: AttributesFormatString=Saturate: %<SaturateOnIntegerOverflow>
  Add1 : Sum  InitFcn=|  Inputs=+-  OutDataTypeStr=int32  SaturateOnIntegerOverflow=on  InputSameDT=on
      | if(exist('MBDS_BlockCallback', 'file'))
      |    MBDS_BlockCallback('Update', gcb);  
      | end
      settings: AttributesFormatString=Saturate: %<SaturateOnIntegerOverflow>
  Constant : Constant  InitFcn=|  OutDataTypeStr=Inherit: Inherit via back propagation
      | if(exist('MBDS_BlockCallback', 'file'))
      |    MBDS_BlockCallback('Update', gcb);  
      | end
  Constant1 : Constant  InitFcn=|  OutDataTypeStr=Inherit: Inherit via back propagation
      | if(exist('MBDS_BlockCallback', 'file'))
      |    MBDS_BlockCallback('Update', gcb);  
      | end
  LE1 : Subsystem  InitFcn=|  mask(LE){MBDS_LibraryBlock=on, InputSameDT=on, MBDS_BlockVersion=05.20}
      | if(exist('MBDS_BlockCallback', 'file'))
      |    MBDS_BlockCallback('Update', gcb);
      | end
      mask prompts: MBDS_LibraryBlock "MBDS library block"; InputSameDT "Require all inputs to have the same data type"; MBDS_BlockVersion "Block version:"
      mask help: The block compares if the first input signal is lower than or equal to the second input signal.
      mask init: same as APP_MyApplication/Model/APP_MyApplication_/OR
      mask Help: eval(['open([workdir(''library_dir:''),''\Blockset\help\'',get_param(gcb,''MaskType''),''.html''])'])
      mask Callback InputSameDT:
      | % Adopt value
      | if(exist('MBDS_BlockCallback', 'file'))
      |    MBDS_BlockCallback('InputSameDT', gcb);
      | end
      mask DialogControl ParameterTabVar0 Prompt: Signal Attributes
      mask DialogControl ParameterTabVar01 Prompt: Version
      mask Display:
      | % Show icon or block text
      | if(exist('MBDS_BlockCallback', 'file'))
      |    image(imread('LE.tif','tif'),[0.33,0.33,0.37,0.37])
      |    disp('')
      | else
      |    disp(sprintf('<='));
      | end
  LE2 : Subsystem  InitFcn=|  mask(LE){MBDS_LibraryBlock=on, InputSameDT=on, MBDS_BlockVersion=05.20}
      | if(exist('MBDS_BlockCallback', 'file'))
      |    MBDS_BlockCallback('Update', gcb);
      | end
      mask prompts: MBDS_LibraryBlock "MBDS library block"; InputSameDT "Require all inputs to have the same data type"; MBDS_BlockVersion "Block version:"
      mask help: The block compares if the first input signal is lower than or equal to the second input signal.
      mask init: same as APP_MyApplication/Model/APP_MyApplication_/OR
      mask Help: eval(['open([workdir(''library_dir:''),''\Blockset\help\'',get_param(gcb,''MaskType''),''.html''])'])
      mask Callback InputSameDT:
      | % Adopt value
      | if(exist('MBDS_BlockCallback', 'file'))
      |    MBDS_BlockCallback('InputSameDT', gcb);
      | end
      mask DialogControl ParameterTabVar0 Prompt: Signal Attributes
      mask DialogControl ParameterTabVar01 Prompt: Version
      mask Display:
      | % Show icon or block text
      | if(exist('MBDS_BlockCallback', 'file'))
      |    image(imread('LE.tif','tif'),[0.33,0.33,0.37,0.37])
      |    disp('')
      | else
      |    disp(sprintf('<='));
      | end
  Mux : Mux  InitFcn=|  Inputs=2
      | try
      |    MBDS_BlockCallback('Update', gcb);
      | end
  Mux1 : Mux  InitFcn=|  Inputs=2
      | try
      |    MBDS_BlockCallback('Update', gcb);
      | end
  OutputsBusSelector : BusSelector  InitFcn=|  OutputSignals=bo_Out1,i32_Out2
      | try                                  
      |    MBDS_BlockCallback('Update', gcb);
      | end
  ReferencesBusSelector : BusSelector  InitFcn=|  OutputSignals=bo_Out1_Ref,i32_Out2_Ref
      | try                                  
      |    MBDS_BlockCallback('Update', gcb);
      | end
  Signal_Inspection1 : Scope  NumInputPorts=2
  Visual_Inspection2 : Scope  NumInputPorts=2
  bo_IsOutputValid : Outport  InitFcn=|  PortDimensions=1
      | try
      |    MBDS_BlockCallback('Update', gcb);
      | end
  wires:
  LE2/1(y) -> AND/1(u1)
  AND/1(y) -> bo_IsOutputValid/1
  Constant/1 -> LE2/2(u2)
  Abs2/1 -> LE2/1(u1)
  Constant1/1 -> LE1/2(u2)
  Abs1/1 -> LE1/1(u1)
  LE1/1(y) -> AND/2(u2)
  Add1/1 -> Visual_Inspection2/2, Abs1/1  "i32_Error"
  Mux1/1 -> Visual_Inspection2/1
  Add/1 -> Signal_Inspection1/2, Abs2/1  "i32_Error"
  ReferencesBusSelector/1 -> Add/2, Mux/2  "<bo_Out1_Ref>"
  ReferencesBusSelector/2 -> Add1/2, Mux1/2  "<i32_Out2_Ref>"
  Mux/1 -> Signal_Inspection1/1
  OutputsBusSelector/1 -> Add/1, Mux/1  "<bo_Out1>"
  OutputsBusSelector/2 -> Add1/1, Mux1/1  "<i32_Out2>"
  st_Outputs/1 -> OutputsBusSelector/1
  st_References/1 -> ReferencesBusSelector/1

== system APP_MyApplication/Outputs/References ==
  Demux : Demux  Tag=STV Demux  InitFcn=|  Outputs=2
      | try
      |    MBDS_BlockCallback('Update', gcb);
      | end
  FromWs : FromWorkspace  Tag=STV FromWs  VariableName=tuvar  OutputAfterFinalValue=Holding final value
      SigBuilderData=|
      | common.afterFinalStr = 'Hold final value'
      | common.sampleTime = '-1'
      | dataSet(1).timeRange = [0 10]
      | dataSet(1).name = 'Common Test'
      | dataSet(2).timeRange = [0 10]
      | dataSet(2).name = 'TC1'
      | dataSet(3).timeRange = [0 10]
      | dataSet(3).name = 'TC2'
      | sbobj.Groups(1).Name = 'Common Test'
      | sbobj.Groups(1).Signals(1).Name = 'bo_Out1_Ref'
      | sbobj.Groups(1).Signals(1).XData = [0 2 2 8 8 10]
      | sbobj.Groups(1).Signals(1).YData = [0 0 1 1 0 0]
      | sbobj.Groups(1).Signals(2).Name = 'i32_Out2_Ref'
      | sbobj.Groups(1).Signals(2).XData = [0 10]
      | sbobj.Groups(1).Signals(2).YData = [0 10000]
      | sbobj.Groups(2).Name = 'TC1'
      | sbobj.Groups(2).Signals(1).Name = 'bo_Out1_Ref'
      | sbobj.Groups(2).Signals(1).XData = [0 2 2 8 8 10]
      | sbobj.Groups(2).Signals(1).YData = [0 0 1 1 0 0]
      | sbobj.Groups(2).Signals(2).Name = 'i32_Out2_Ref'
      | sbobj.Groups(2).Signals(2).XData = [0 10]
      | sbobj.Groups(2).Signals(2).YData = [0 10000]
      | sbobj.Groups(3).Name = 'TC2'
      | sbobj.Groups(3).Signals(1).Name = 'bo_Out1_Ref'
      | sbobj.Groups(3).Signals(1).XData = [0 2 2 8 8 10]
      | sbobj.Groups(3).Signals(1).YData = [0 0 1 1 0 0]
      | sbobj.Groups(3).Signals(2).Name = 'i32_Out2_Ref'
      | sbobj.Groups(3).Signals(2).XData = [0 10]
      | sbobj.Groups(3).Signals(2).YData = [0 10000]
  bo_Out1_Ref : Outport  Tag=STV Outport
  i32_Out2_Ref : Outport  Tag=STV Outport  Port=2
  wires:
  Demux/1 -> bo_Out1_Ref/1
  FromWs/1 -> Demux/1
  Demux/2 -> i32_Out2_Ref/1

== system APP_MyApplication/Stimuli/Stimuli ==
  Demux : Demux  Tag=STV Demux  InitFcn=|  Outputs=2
      | try
      |    MBDS_BlockCallback('Update', gcb);
      | end
  FromWs : FromWorkspace  Tag=STV FromWs  VariableName=tuvar  OutputAfterFinalValue=Holding final value
      SigBuilderData=|
      | common.afterFinalStr = 'Hold final value'
      | common.sampleTime = '-1'
      | dataSet(1).timeRange = [0 10]
      | dataSet(1).name = 'Common Test'
      | dataSet(2).timeRange = [0 10]
      | dataSet(2).name = 'TC1'
      | dataSet(3).timeRange = [0 10]
      | dataSet(3).name = 'TC2'
      | sbobj.Groups(1).Name = 'Common Test'
      | sbobj.Groups(1).Signals(1).Name = 'bo_In1'
      | sbobj.Groups(1).Signals(1).XData = [0 2 2 8 8 10]
      | sbobj.Groups(1).Signals(1).YData = [0 0 1 1 0 0]
      | sbobj.Groups(1).Signals(2).Name = 'i32_In2'
      | sbobj.Groups(1).Signals(2).XData = [0 10]
      | sbobj.Groups(1).Signals(2).YData = [0 10000]
      | sbobj.Groups(2).Name = 'TC1'
      | sbobj.Groups(2).Signals(1).Name = 'bo_In1'
      | sbobj.Groups(2).Signals(1).XData = [0 2 2 8 8 10]
      | sbobj.Groups(2).Signals(1).YData = [0 0 1 1 0 0]
      | sbobj.Groups(2).Signals(2).Name = 'i32_In2'
      | sbobj.Groups(2).Signals(2).XData = [0 10]
      | sbobj.Groups(2).Signals(2).YData = [0 10000]
      | sbobj.Groups(3).Name = 'TC2'
      | sbobj.Groups(3).Signals(1).Name = 'bo_In1'
      | sbobj.Groups(3).Signals(1).XData = [0 2 2 8 8 10]
      | sbobj.Groups(3).Signals(1).YData = [0 0 1 1 0 0]
      | sbobj.Groups(3).Signals(2).Name = 'i32_In2'
      | sbobj.Groups(3).Signals(2).XData = [0 10]
      | sbobj.Groups(3).Signals(2).YData = [0 10000]
  bo_In1 : Outport  Tag=STV Outport
  i32_In2 : Outport  Tag=STV Outport  Port=2
  wires:
  Demux/1 -> bo_In1/1
  FromWs/1 -> Demux/1
  Demux/2 -> i32_In2/1

== system APP_MyApplication/Model/APP_MyApplication_/A-CAN(2) ==
  Constant1 : Constant  InitFcn=|  OutDataTypeStr=boolean
      | if(exist('MBDS_BlockCallback', 'file'))
      |    MBDS_BlockCallback('Update', gcb);  
      | end
  Constant2 : Constant  InitFcn=|  OutDataTypeStr=boolean
      | if(exist('MBDS_BlockCallback', 'file'))
      |    MBDS_BlockCallback('Update', gcb);  
      | end
  Constant3 : Constant  InitFcn=|  Value=2  OutDataTypeStr=uint8
      | if(exist('MBDS_BlockCallback', 'file'))
      |    MBDS_BlockCallback('Update', gcb);  
      | end
  in_IN_ACAN.TX_Gen.ACAN_TX_01.MessageState : KIBES_Signal/KIBES_Signal  MBDS_LibraryBlock=on  DatabaseKey=84  SignalName=IN_ACAN.TX_Gen.ACAN_TX_01.MessageState  SymbolName=IN_ACAN_TX_Gen_ACAN_TX_01_MessageState_000084  DataType=uint16  Init=0  Slope=1  Bias=0  DataSize=1  fpDataType=uint16  BlockIOType=Inport  DeviceType=0
  out_ACAN.GenericGatewayMessage.MessageEnable : KIBES_Signal/KIBES_Signal  MBDS_LibraryBlock=on  DatabaseKey=549  SignalName=ACAN.GenericGatewayMessage.MessageEnable  SymbolName=ACAN_GenericGatewayMessage_MessageEnable_000549  DataType=boolean  Init=0  Slope=1  Bias=0  DataSize=1  fpDataType=boolean  BlockIOType=Outport  DeviceType=0
  out_OUT_ACAN.TX_Gen.ACAN_TX_01.MessageEnable : KIBES_Signal/KIBES_Signal  MBDS_LibraryBlock=on  DatabaseKey=83  SignalName=OUT_ACAN.TX_Gen.ACAN_TX_01.MessageEnable  SymbolName=OUT_ACAN_TX_Gen_ACAN_TX_01_MessageEnable_000083  DataType=boolean  Init=0  Slope=1  Bias=0  DataSize=1  fpDataType=boolean  BlockIOType=Outport  DeviceType=0
  out_OUT_ACAN.TX_Gen.ACAN_TX_01.Val1 : KIBES_Signal/KIBES_Signal  MBDS_LibraryBlock=on  DatabaseKey=85  SignalName=OUT_ACAN.TX_Gen.ACAN_TX_01.Val1  SymbolName=OUT_ACAN_TX_Gen_ACAN_TX_01_Val1_000085  DataType=uint8  Init=0  Slope=1  Bias=0  DataSize=1  fpDataType=uint8  BlockIOType=Outport  DeviceType=0
  wires:
  Constant3/1 -> out_OUT_ACAN.TX_Gen.ACAN_TX_01.Val1/1
  Constant1/1 -> out_OUT_ACAN.TX_Gen.ACAN_TX_01.MessageEnable/1
  Constant2/1 -> out_ACAN.GenericGatewayMessage.MessageEnable/1

== system APP_MyApplication/Model/APP_MyApplication_/Accelerometer  ==
  in_InertianSensorDevice.AccelerometerSubdevice.Ax : KIBES_Signal/KIBES_Signal  MBDS_LibraryBlock=on  DatabaseKey=651  SignalName=InertianSensorDevice.AccelerometerSubdevice.Ax  SymbolName=InertianSensorDevice_AccelerometerSubdevice_Ax_000651  DataType=int16  Init=0  Slope=1  Bias=0  DataSize=1  fpDataType=int16  BlockIOType=Inport  DeviceType=0
  in_InertianSensorDevice.AccelerometerSubdevice.Ay : KIBES_Signal/KIBES_Signal  MBDS_LibraryBlock=on  DatabaseKey=652  SignalName=InertianSensorDevice.AccelerometerSubdevice.Ay  SymbolName=InertianSensorDevice_AccelerometerSubdevice_Ay_000652  DataType=int16  Init=0  Slope=1  Bias=0  DataSize=1  fpDataType=int16  BlockIOType=Inport  DeviceType=0
  in_InertianSensorDevice.AccelerometerSubdevice.Az : KIBES_Signal/KIBES_Signal  MBDS_LibraryBlock=on  DatabaseKey=650  SignalName=InertianSensorDevice.AccelerometerSubdevice.Az  SymbolName=InertianSensorDevice_AccelerometerSubdevice_Az_000650  DataType=int16  Init=0  Slope=1  Bias=0  DataSize=1  fpDataType=int16  BlockIOType=Inport  DeviceType=0
  in_InertianSensorDevice.AccelerometerSubdevice.DeviceState : KIBES_Signal/KIBES_Signal  MBDS_LibraryBlock=on  DatabaseKey=653  SignalName=InertianSensorDevice.AccelerometerSubdevice.DeviceState  SymbolName=InertianSensorDevice_AccelerometerSubdevice_DeviceState_000653  DataType=uint16  Init=0  Slope=1  Bias=0  DataSize=1  fpDataType=uint16  BlockIOType=Inport  DeviceType=0
  in_STIMD.Accel_Enable : KIBES_Signal/KIBES_Signal  MBDS_LibraryBlock=on  DatabaseKey=654  SignalName=STIMD.Accel_Enable  SymbolName=STIMD_Accel_Enable_000654  DataType=boolean  Init=0  Slope=1  Bias=0  DataSize=1  fpDataType=boolean  BlockIOType=Inport  DeviceType=2
  out_InertianSensorDevice.AccelerometerSubdevice.DeviceEnable : KIBES_Signal/KIBES_Signal  MBDS_LibraryBlock=on  DatabaseKey=649  SignalName=InertianSensorDevice.AccelerometerSubdevice.DeviceEnable  SymbolName=InertianSensorDevice_AccelerometerSubdevice_DeviceEnabl_000649  DataType=boolean  Init=0  Slope=1  Bias=0  DataSize=1  fpDataType=boolean  BlockIOType=Outport  DeviceType=0
  wires:
  in_STIMD.Accel_Enable/1 -> out_InertianSensorDevice.AccelerometerSubdevice.DeviceEnable/1

== system APP_MyApplication/Model/APP_MyApplication_/AnalogIn ==
